simulink model "filtertest"  (Simulink 6.1)
settings: Solver=ode45  StartTime=0.0  StopTime=10.0  RelTol=1e-3
undefined symbols (not defined in the file or in its folder): ww, zz
libraries: simulink x1
settings Model: LastModifiedBy=fhuang
settings DebuggingCC: SolverPrmCheckMsg=warning

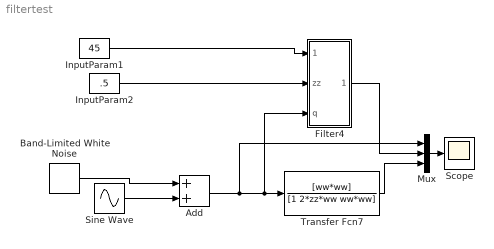
== system filtertest ==
  Add : Sum  OutScaling=2^-10
  Band-Limited White Noise : simulink/Sources/Band-Limited White Noise  Cov=[0.001]  Ts=.001  seed=[23341]
  Filter4 : Subsystem
  InputParam1 : Constant  Value=45
  InputParam2 : Constant  Value=.5
  Mux : Mux  Inputs=3
  Scope : Scope
  Sine Wave : Sin  Amplitude=10  SampleTime=0
  Transfer Fcn7 : TransferFcn  Numerator=[ww*ww]  Denominator=[1 2*zz*ww ww*ww]
  wires:
  InputParam1/1 -> Filter4/1(ww)
  InputParam2/1 -> Filter4/2(zz)
  Add/1 -> Filter4/3(q), Transfer Fcn7/1, Mux/1
  Mux/1 -> Scope/1
  Transfer Fcn7/1 -> Mux/3
  Band-Limited White Noise/1 -> Add/1
  Sine Wave/1 -> Add/2
  Filter4/1(q_filt) -> Mux/2

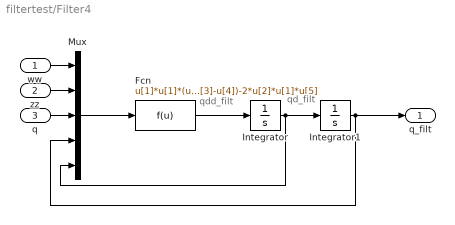
== system filtertest/Filter4 ==
  note: qd_filt
  note: qdd_filt
  ww : Inport  Port=1  LatchInput=off
  zz : Inport  Port=2  LatchInput=off
  q : Inport  Port=3  LatchInput=off
  Fcn : Fcn  Expr=u[1]*u[1]*(u[3]-u[4])-2*u[2]*u[1]*u[5]
  Integrator : Integrator
  Integrator1 : Integrator
  Mux : Mux  Inputs=5
  q_filt : Outport
  wires:
  q/1 -> Mux/3
  zz/1 -> Mux/2
  Integrator1/1 -> Mux/4, q_filt/1
  ww/1 -> Mux/1
  Mux/1 -> Fcn/1
  Fcn/1 -> Integrator/1
  Integrator/1 -> Mux/5, Integrator1/1
